simulink model "my_LUT"  (R2025b)
settings: Solver=FixedStepAuto  StartTime=0.0  StopTime=10.0  RelTol=1e-3
undefined symbols (not defined in the file or in its folder): xx, yy
libraries: simulink x1
settings Model: Creator=Huawei  LastModifiedBy=Huawei
settings OptimizationCC: UseDivisionForNetSlopeComputation=on

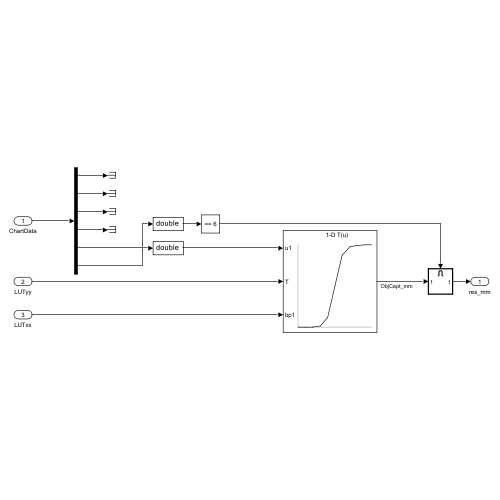
[thumbnail: Simulink's stored preview of the top-level diagram]
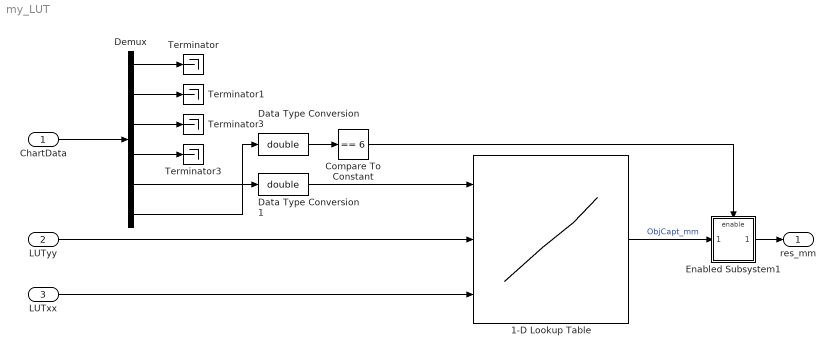
== system my_LUT ==
  ChartData : Inport  OutDataTypeStr=single  PortDimensions=6
  LUTyy : Inport  Port=2  OutDataTypeStr=double  PortDimensions=[1 25]
  LUTxx : Inport  Port=3  OutDataTypeStr=double  PortDimensions=[1 25]
  1-D Lookup Table : Lookup_n-D  NumberOfTableDimensions=1  LookupTableObject=myLUTobj  BreakpointsForDimension1Source=Input port  BreakpointsForDimension1=xx  IndexSearchMethod=Linear search  TableSource=Input port  Table=yy  InternalRulePriority=Speed  RndMeth=Simplest
      settings: InputPortMap=u0,p221,p5
  Compare To Constant : simulink/Logic and Bit Operations/Compare To Constant  relop===  const=6  OutDataTypeStr=boolean
  Data Type Conversion1 : DataTypeConversion  OutDataTypeStr=double  SaturateOnIntegerOverflow=off  RndMeth=Floor
  Data Type Conversion3 : DataTypeConversion  OutDataTypeStr=double  SaturateOnIntegerOverflow=off  RndMeth=Floor
  Demux : Demux  Outputs=6
  Enabled Subsystem1 : Subsystem  TreatAsAtomicUnit=on
  Terminator{,1..3} (4 alike) : Terminator
  res_mm : Outport  OutDataTypeStr=double  PortDimensions=1
  wires:
  Demux/6 -> Data Type Conversion3/1
  Demux/5 -> Data Type Conversion1/1
  Compare To Constant/1 -> Enabled Subsystem1/Enable
  LUTyy/1 -> 1-D Lookup Table/2
  Data Type Conversion1/1 -> 1-D Lookup Table/1
  Data Type Conversion3/1 -> Compare To Constant/1
  LUTxx/1 -> 1-D Lookup Table/3
  ChartData/1 -> Demux/1
  Demux/1 -> Terminator/1
  Demux/2 -> Terminator1/1
  Demux/3 -> Terminator2/1
  Demux/4 -> Terminator3/1
  1-D Lookup Table/1 -> Enabled Subsystem1/1(In1)  "ObjCapt_mm"
  Enabled Subsystem1/1(Out1) -> res_mm/1

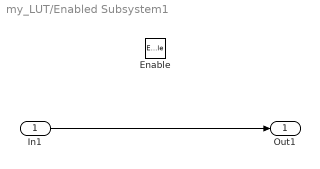
== system my_LUT/Enabled Subsystem1 ==
  In1 : Inport
  Enable : EnablePort
  Out1 : Outport
  wires:
  In1/1 -> Out1/1
